simulink model "Ejercicio3_13_03_17"  (R2013a)
settings: Solver=ode45  StartTime=0.0  StopTime=10.0  RelTol=1e-3
libraries: powerlib x24, powerlib_meascontrol x1
settings Model: Creator=Miguel  LastModifiedBy=Miguel

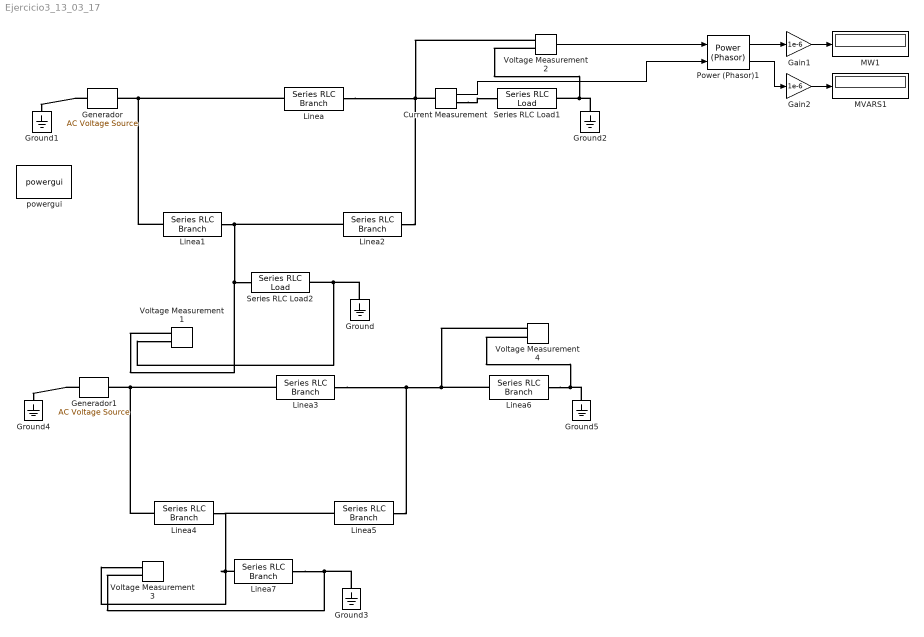
== system Ejercicio3_13_03_17 ==
  Current Measurement : powerlib/Measurements/Current Measurement  PhasorSimulation=on  OutputType=Complex  PSBequivalent=0
  Gain1 : Gain  Gain=1e-6
  Gain2 : Gain  Gain=1e-6
  Generador : powerlib/Electrical Sources/AC Voltage Source  Amplitude=3.15e5*sqrt(2)  Phase=0  Frequency=60  SampleTime=0  Measurements=None
  Generador1 : powerlib/Electrical Sources/AC Voltage Source  Amplitude=3.15e5*sqrt(2)  Phase=0  Frequency=60  SampleTime=0  Measurements=None
  Ground{,1..5} (6 alike) : powerlib/Elements/Ground  LConnTagsString=a
  Linea : powerlib/Elements/Series RLC Branch  LConnTagsString=__new0  RConnTagsString=__new0  BranchType=RL  Resistance=0.02*900  Inductance=0.04*900/(2*pi*60)  SetiL0=off  InitialCurrent=0  Capacitance=1e-6  Setx0=off  InitialVoltage=0  Measurements=None
  Linea1 : powerlib/Elements/Series RLC Branch  LConnTagsString=__new0  RConnTagsString=__new0  BranchType=RL  Resistance=0.01*900  Inductance=0.03*900/(2*pi*60)  SetiL0=off  InitialCurrent=0  Capacitance=1e-6  Setx0=off  InitialVoltage=0  Measurements=None
  Linea2 : powerlib/Elements/Series RLC Branch  LConnTagsString=__new0  RConnTagsString=__new0  BranchType=RL  Resistance=0.0125*900  Inductance=0.025*900/(2*pi*60)  SetiL0=off  InitialCurrent=0  Capacitance=1e-6  Setx0=off  InitialVoltage=0  Measurements=None
  Linea3 : powerlib/Elements/Series RLC Branch  LConnTagsString=__new0  RConnTagsString=__new0  BranchType=RL  Resistance=0.02*900  Inductance=0.04*900/(2*pi*60)  SetiL0=off  InitialCurrent=0  Capacitance=1e-6  Setx0=off  InitialVoltage=0  Measurements=None
  Linea4 : powerlib/Elements/Series RLC Branch  LConnTagsString=__new0  RConnTagsString=__new0  BranchType=RL  Resistance=0.01*900  Inductance=0.03*900/(2*pi*60)  SetiL0=off  InitialCurrent=0  Capacitance=1e-6  Setx0=off  InitialVoltage=0  Measurements=None
  Linea5 : powerlib/Elements/Series RLC Branch  LConnTagsString=__new0  RConnTagsString=__new0  BranchType=RL  Resistance=0.0125*900  Inductance=0.025*900/(2*pi*60)  SetiL0=off  InitialCurrent=0  Capacitance=1e-6  Setx0=off  InitialVoltage=0  Measurements=None
  Linea6 : powerlib/Elements/Series RLC Branch  LConnTagsString=__new0  RConnTagsString=__new0  BranchType=RL  Resistance=285.4625564  Inductance=122.5953769/(2*pi*60)  SetiL0=off  InitialCurrent=0  Capacitance=1e-6  Setx0=off  InitialVoltage=0  Measurements=None
  Linea7 : powerlib/Elements/Series RLC Branch  LConnTagsString=__new0  RConnTagsString=__new0  BranchType=RL  Resistance=587.9858516  Inductance=191.7529617/(2*pi*60)  SetiL0=off  InitialCurrent=0  Capacitance=1e-6  Setx0=off  InitialVoltage=0  Measurements=None
  MVARS1 : Display
  MW1 : Display
  Power (Phasor)1 : powerlib_meascontrol/Measurements/Power (Phasor)
  Series RLC Load1 : powerlib/Elements/Series RLC Load  LConnTagsString=a  RConnTagsString=__new0  NominalVoltage=2.9455e5  NominalFrequency=60  ActivePower=256.6e6  InductivePower=110.2e6  CapacitivePower=0  Setx0=off  InitialVoltage=0  SetiL0=off  InitialCurrent=0  Measurements=None
  Series RLC Load2 : powerlib/Elements/Series RLC Load  LConnTagsString=a  RConnTagsString=__new0  NominalVoltage=3.0027e5  NominalFrequency=60  ActivePower=138.6e6  InductivePower=45.2e6  CapacitivePower=0  Setx0=off  InitialVoltage=0  SetiL0=off  InitialCurrent=0  Measurements=None
  Voltage Measurement{1..4} (4 alike) : powerlib/Measurements/Voltage Measurement  PhasorSimulation=on  OutputType=Complex  PSBequivalent=0
  powergui : powerlib/powergui  Priority=1  SimulationMode=Phasor  SolverType=Tustin  SampleTime=50e-6  frequency=60  SPID=off  DisableSnubberDevices=off  DisableRonSwitches=off  DisableVfSwitches=off  SwTol=0  Interpol=off  DisplayEquations=off  frequencyindice=60  Pbase=100e6  ErrMax=1e-4  Iterations=50  UnitsV=kV  UnitsW=MW  FunctionMessages=off  echomessages=off  HookPort=off  EnableUseOfTLC=off  x0status=blocks  RestoreLinks=warning  ResistiveCurrentMeasurement=off  Frange=[0:2:500]  Ylog=off  Xlog=on  ShowGrid=off  save=off  variable=ZData  ZoomFFT=off  StartTime=0.0  cycles=1  DisplayStyle=1  fundamental=60  FreqAxis=off  MaxFrequency=1000  frequencyindicesteady=1  RmsSteady=2  display=off  Ts=0  methode=off
  wires:
  Power (Phasor)1/1 -> Gain1/1
  Power (Phasor)1/2 -> Gain2/1
  Gain1/1 -> MW1/1
  Gain2/1 -> MVARS1/1
  Current Measurement/1 -> Power (Phasor)1/2
  Voltage Measurement2/1 -> Power (Phasor)1/1
  connections:
  Linea/LConn1 -- Linea1/LConn1 -- Generador/RConn1
  Linea/RConn1 -- Linea2/RConn1 -- Current Measurement/LConn1 -- Voltage Measurement2/LConn1
  Linea2/LConn1 -- Linea1/RConn1 -- Voltage Measurement1/LConn1 -- Series RLC Load2/LConn1
  Ground/LConn1 -- Voltage Measurement1/LConn2 -- Series RLC Load2/RConn1
  Generador/LConn1 -- Ground1/LConn1
  Ground2/LConn1 -- Voltage Measurement2/LConn2 -- Series RLC Load1/RConn1
  Linea3/LConn1 -- Linea4/LConn1 -- Generador1/RConn1
  Linea5/RConn1 -- Linea6/LConn1 -- Voltage Measurement4/LConn1 -- Linea3/RConn1
  Linea5/LConn1 -- Linea4/RConn1 -- Linea7/LConn1 -- Voltage Measurement3/LConn1
  Ground3/LConn1 -- Linea7/RConn1 -- Voltage Measurement3/LConn2
  Ground5/LConn1 -- Linea6/RConn1 -- Voltage Measurement4/LConn2
  Generador1/LConn1 -- Ground4/LConn1
  Current Measurement/RConn1 -- Series RLC Load1/LConn1
